simulink model "MSFartoystyringSurgeBoi"  (R2017b)
settings: Solver=ode45  StartTime=tstart  StopTime=tstop  RelTol=1e-3  EnableMultiTasking=on
values from neighbouring files (symbols this model uses):
  c = 0    [test_surge_boi.m]
  nc_step = 4    [test_surge_boi.m]
  p0 = zeros(2,1)    [test_surge_boi.m]
  psi0 = 0    [test_surge_boi.m]
  r0 = 0    [test_surge_boi.m]
  tsamp = 10    [test_surge_boi.m]
  v0 = [0.00000001 0]'    [test_surge_boi.m]
undefined symbols (not defined in the file or in its folder): msfartoystyring
settings Model: ExtModeAutoUpdateStatusClock=off  Creator=christh  LastModifiedBy=sigtot
settings DataIOCC: LimitDataPoints=on  SaveFormat=Array  SignalLoggingSaveFormat=ModelDataLogs
settings OptimizationCC: ExpressionDepthLimit=2147483647  InitFltsAndDblsToZero=on  LifeSpan=inf
settings DebuggingCC: UnderspecifiedInitializationDetection=Classic  MergeDetectMultiDrivingBlocksExec=none  SolverPrmCheckMsg=warning  FcnCallInpInsideContextMsg=warning  StateNameClashWarn=warning  SFUnexpectedBacktrackingDiag=warning  SFNoUnconditionalDefaultTransitionDiag=warning
settings HardwareCC: ProdBitPerPointer=32  ProdBitPerSizeT=32  ProdBitPerPtrDiffT=32  ProdLargestAtomicFloat=None  ProdIntDivRoundTo=Undefined  ProdEndianess=Unspecified  ProdWordSize=32  ProdHWDeviceType=32-bit Generic
settings ModelReferenceCC: PropagateSignalLabelsOutOfModel=off
settings CodeAppCC: StateflowObjectComments=on
settings GRTTargetCC: TargetLangStandard=C89/C90 (ANSI)  GeneratePreprocessorConditionals=Disable all  CombineOutputUpdateFcns=off  GRTInterface=on
settings ConfigComp: CovMetricSettings=dw  CovHtmlReporting=on  CovSaveCumulativeToWorkspaceVar=on  CovSaveSingleToWorkspaceVar=on  CovExternalEMLEnable=off

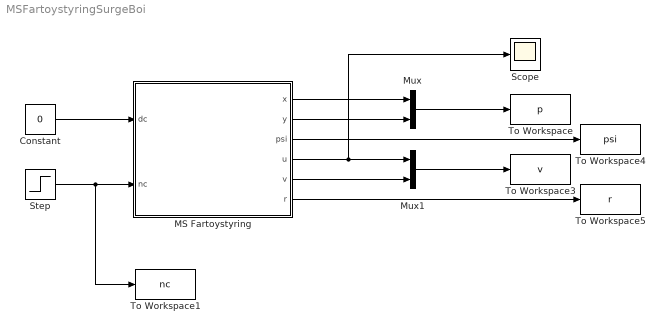
== system MSFartoystyringSurgeBoi ==
  Constant : Constant  Value=0
  MS Fartoystyring : Subsystem  mask(MS Fartoystyring for Assignment 3 G&C){x0=p0(1), y0=p0(2), u0=v0(1), v0=v0(2), psi0=psi0, r0=r0, c=c}
      mask prompts: x0 "x(t0) (m)"; y0 "y(t0) (m)"; u0 "u(t0) (m/s)"; v0 "v(t0) (m/s)"; psi0 "psi(t0) (rad)"; r0 "r(t0) (rad/s)"; c "current (0 or 1)"
      mask help:
      | Block corresponding to Figure 1 in the assignment text. Gives the response of the ship.
      |
      | The design speed of MS Fartoystyring is u=8.23 m/s.
      |
      | Input:
      | dc: commanded rudder (rad), dmax=25*pi/180
      | nc: commanded shaft speed (rad/s), nmax=85*2*pi/60
      |
      | Output:
      | x: north pos (m)
      | y: east pos (m)
      | u: surge (m/s)
      | v: sway (m/s)
      | psi: heading (rad)
      | r: yaw (rad/s)
      mask Help: Comments, bugs and help requests can be directed to the TA. Email on course website.
  Mux : Mux  Inputs=2
  Mux1 : Mux  Inputs=2
  Scope : Scope
  Step : Step  After=nc_step  SampleTime=0
  To Workspace : ToWorkspace  VariableName=p  SampleTime=tsamp
  To Workspace1 : ToWorkspace  VariableName=nc  SampleTime=tsamp
  To Workspace3 : ToWorkspace  VariableName=v  SampleTime=tsamp
  To Workspace4 : ToWorkspace  VariableName=psi  SampleTime=tsamp
  To Workspace5 : ToWorkspace  VariableName=r  SampleTime=tsamp
  wires:
  MS Fartoystyring/2(y) -> Mux/2
  MS Fartoystyring/4(u) -> Scope/1, Mux1/1
  MS Fartoystyring/5(v) -> Mux1/2
  Mux/1 -> To Workspace/1
  Mux1/1 -> To Workspace3/1
  MS Fartoystyring/3(psi) -> To Workspace4/1
  MS Fartoystyring/6(r) -> To Workspace5/1
  Constant/1 -> MS Fartoystyring/1(dc)
  MS Fartoystyring/1(x) -> Mux/1
  Step/1 -> To Workspace1/1, MS Fartoystyring/2(nc)

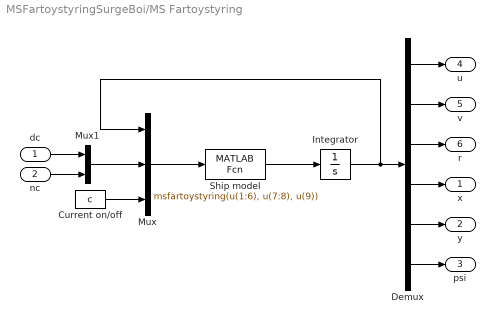
== system MSFartoystyringSurgeBoi/MS Fartoystyring ==
  dc : Inport
  nc : Inport  Port=2
  Current on/off : Constant  Value=c
  Demux : Demux  Outputs=6
  Integrator : Integrator  InitialCondition=[u0 v0 r0 x0 y0 psi0]'
  Mux : Mux  Inputs=3
  Mux1 : Mux  Inputs=2
  Ship model : MATLABFcn  MATLABFcn=msfartoystyring(u(1:6), u(7:8), u(9))  OutputDimensions=6
  x : Outport
  y : Outport  Port=2
  psi : Outport  Port=3
  u : Outport  Port=4
  v : Outport  Port=5
  r : Outport  Port=6
  wires:
  Integrator/1 -> Mux/1, Demux/1
  Mux1/1 -> Mux/2
  dc/1 -> Mux1/1
  nc/1 -> Mux1/2
  Demux/1 -> u/1
  Demux/2 -> v/1
  Demux/3 -> r/1
  Demux/4 -> x/1
  Demux/5 -> y/1
  Demux/6 -> psi/1
  Current on/off/1 -> Mux/3
  Ship model/1 -> Integrator/1
  Mux/1 -> Ship model/1
